simulink library "HX_data_fit"  (Simulink 8.2)
settings: Solver=ode45  StartTime=0.0  StopTime=10.0  RelTol=1e-3
undefined symbols (not defined in the file): dia, height, nodes
libraries: carnot x2
settings Model: Creator=lena.frank  LastModifiedBy=drhf

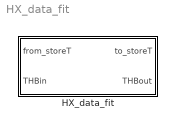
== system HX_data_fit ==
  HX_data_fit : Subsystem  mask(heat exchanger for storage, fitted data){h_in=1, h_out=0, ua0=800, uam=0, uat=0, dplin=100, dpqua=100, nodes=nodes, hgt=height, dia=dia}
      mask prompts: h_in "relative height of inlet"; h_out "relative height of outlet"; ua0 "uac: constant heat transfer coefficient [W/K]"; uam "uam: massflow dependent heat transfer [W*s/(K*kg)]"; uat "uat: temperature difference dependent heat transfer [W/K²]"; dplin "pressure drop linear in mdot [Pa*s/kg]"; dpqua "pressure drop quadratic in mdot [Pa*s²/kg²]"; nodes "Number of nodes (DO NOT CHANGE)"; hgt "Height vector (DO NOT CHANGE)"; dia "Diameter (DO NOT CHANGE)"
      mask help:
      | The block transforms the incoming THV vector to a vector which the storage interprets as a heat exchanger.
      | Give inlet and outlet as a relative position 0=bottom to 1=top
      | The heat transfer is calculated by:
      | UA = uac + mdot*uam + (Theatexchanger-Tstorage)*uat
      mask init:
      | in = zeros(nodes,1);    % vector of length nodes
      | up = in;                % vector of length nodes
      | down = in;              % vector of length nodes
      | 
      | h_in = max(0,h_in);     % no nodes below 0
      | h_out = max(0,h_out);   % no nodes below 0
      | 
      | inlet = round(h_in*(nodes-1))+1;    % inlet position
      | outlet = round(h_out*(nodes-1))+1;  % outlet position
      | hgt = (h_out-h_in)*hgt;
      | in(inlet)=1;
      | 
      | if (h_in < h_out)           % if inlet below outlet
      |     up(inlet:outlet)=1;     % upwards
      | elseif (h_in > h_out)       % else if inlet above outlet
      |     down(outlet:inlet)=1;   % downwards
      | end
      mask Help: web(fullfile(path_carnot('help'),'StoragePorts_HeatExchangerModels.html'),'-helpbrowser')
      mask Display: disp('HX data')

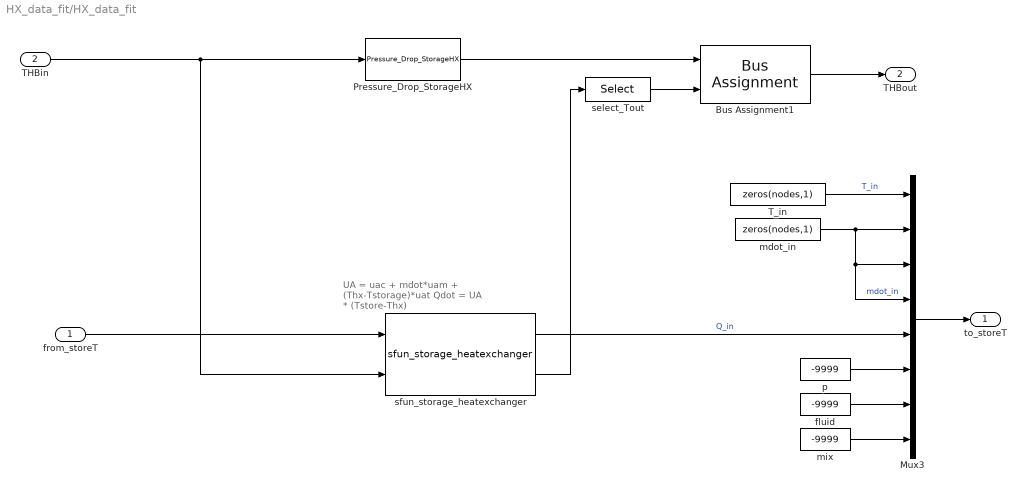
== system HX_data_fit/HX_data_fit ==
  note: UA = uac + mdot*uam + (Thx-Tstorage)*uat
      | Qdot = UA * (Tstore-Thx)
  from_storeT : Inport
  THBin : Inport  Port=2
  Bus Assignment1 : BusAssignment  AssignedSignals=Temperature
  Mux3 : Mux  Inputs=8
  Pressure_Drop_StorageHX : carnot/Basic/Pressure_Drop/Pressure_Drop_StorageHX  dia=dia  hgt=hgt
  T_in : Constant  Value=zeros(nodes,1)
  fluid : Constant  Value=-9999
  mdot_in : Constant  Value=zeros(nodes,1)
  mix : Constant  Value=-9999
  p : Constant  Value=-9999
  select_Tout : Selector  InputPortWidth=nodes  IndexOptions=Index vector (dialog)  Indices=[outlet]  OutputSizes=1
  sfun_storage_heatexchanger : carnot/Basic/Thermal_Models/sfun_storage_heatexchanger  idn=heat transfer from data fit  nodes=nodes  inlet=inlet  outlet=outlet  pp=[ua0, uam, uat, 0,0,0,0]
  to_storeT : Outport
  THBout : Outport  Port=2
  wires:
  Pressure_Drop_StorageHX/1 -> Bus Assignment1/1
  from_storeT/1 -> sfun_storage_heatexchanger/1
  THBin/1 -> sfun_storage_heatexchanger/2, Pressure_Drop_StorageHX/1
  mdot_in/1 -> Mux3/2, Mux3/3, Mux3/4  "mdot_in"
  Mux3/1 -> to_storeT/1
  select_Tout/1 -> Bus Assignment1/2
  T_in/1 -> Mux3/1  "T_in"
  sfun_storage_heatexchanger/1 -> Mux3/5  "Q_in"
  Bus Assignment1/1 -> THBout/1
  p/1 -> Mux3/6
  fluid/1 -> Mux3/7
  mix/1 -> Mux3/8
  sfun_storage_heatexchanger/2 -> select_Tout/1
